simulink model "plant_backup"  (R2026a)
settings: Solver=FixedStepAuto  FixedStep=1e-3
settings Model: DataDictionary=plantParams.sldd  PauseTimes=1  Creator=maxhu  LastModifiedBy=nathanscott

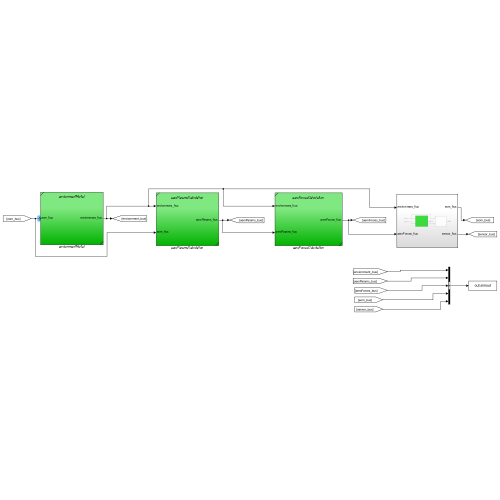
[thumbnail: Simulink's stored preview of the top-level diagram]
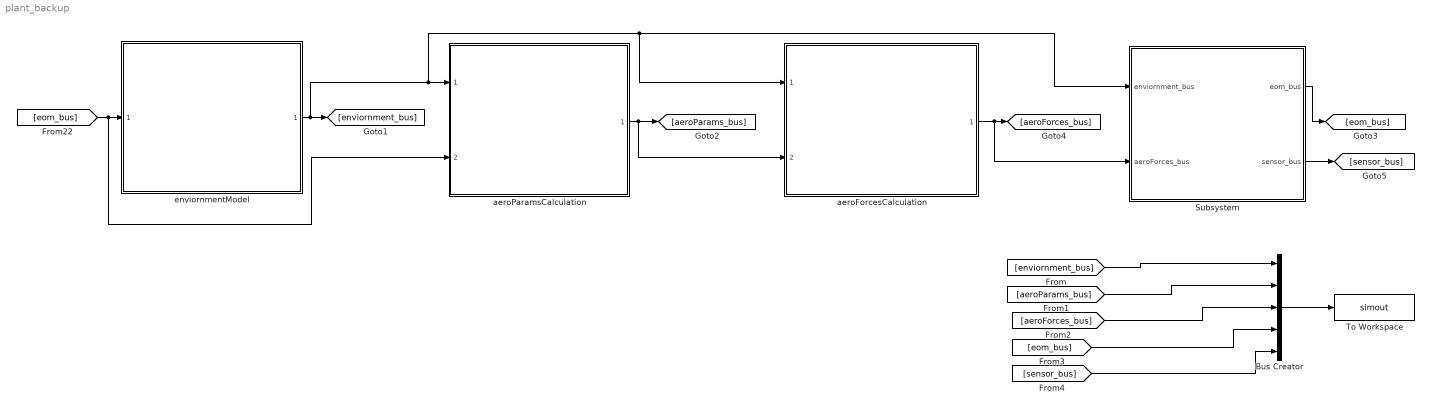
== system plant_backup ==
  Bus Creator : BusCreator  Inputs=5
  Subsystem : Subsystem
  To Workspace : ToWorkspace  VariableName=simout  SaveFormat=Timeseries  SampleTime=-1
  aeroForcesCalculation : Subsystem  ReferencedSubsystem=aeroForcesCalculation
  aeroParamsCalculation : Subsystem  ReferencedSubsystem=aeroParamsCalculation
  enviornmentModel : Subsystem  ReferencedSubsystem=enviornmentModel
  wires:
  Bus Creator/1 -> To Workspace/1
  [eom_bus] -> aeroParamsCalculation/2, enviornmentModel/1
  aeroParamsCalculation/1 -> aeroForcesCalculation/2, [aeroParams_bus]
  enviornmentModel/1 -> [enviornment_bus], Subsystem/1(enviornment_bus), aeroForcesCalculation/1, aeroParamsCalculation/1
  aeroForcesCalculation/1 -> Subsystem/2(aeroForces_bus), [aeroForces_bus]
  [eom_bus] -> Bus Creator/4
  [aeroForces_bus] -> Bus Creator/3
  [aeroParams_bus] -> Bus Creator/2
  [enviornment_bus] -> Bus Creator/1
  Subsystem/1(eom_bus) -> [eom_bus]
  Subsystem/2(sensor_bus) -> [sensor_bus]
  [sensor_bus] -> Bus Creator/5

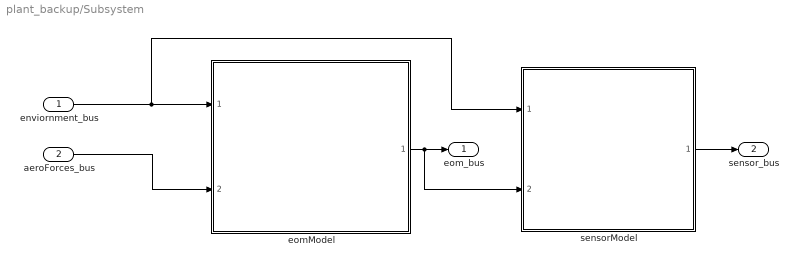
== system plant_backup/Subsystem ==
  enviornment_bus : Inport
  aeroForces_bus : Inport  Port=2
  eomModel : Subsystem  ReferencedSubsystem=eomModel
  sensorModel : Subsystem  ReferencedSubsystem=sensorModels
  eom_bus : Outport
  sensor_bus : Outport  Port=2
  wires:
  aeroForces_bus/1 -> eomModel/2
  enviornment_bus/1 -> eomModel/1, sensorModel/1
  eomModel/1 -> sensorModel/2, eom_bus/1
  sensorModel/1 -> sensor_bus/1
